simulink model "F_mod_A_mod_gsyn_top_trig_mism_sub_simplified"  (R2022a)
settings: Solver=ode15s  StartTime=0.0  StopTime=10  FixedStep=2.5e-4  MaxStep=5e-2  MinStep=1e-5  RelTol=1e-2  AbsTol=1e-2
model workspace (MAT data in the model file):
  base_gsm = 2.3
  base_gsyn = -2
  cos_amp = 2.5
  cos_center = 0
  friction_factor = 1
  mass_density = 951
  mass_radius = 0.05
  mod_strength_gsm = 1.8
  mod_strength_gsyn = 1.8
  noisePwr = 3e-06
  pendulum_length = 0.4267
  prob_event_loss = 0
  ref_angle = 2
  rel_diff = 0.1
  rel_mod = 100000
  rel_noise = 4
  sampleTime = 0.001
  sin_amp = 2.5
  sin_center = 0
  start_angle = 0
  timescale = 0.004
  torque_max = 0.6
settings Model: SimulationMode=accelerator  Creator=chris  LastModifiedBy=chris
settings SolverCC: MaxConsecutiveZCs=10  MaxConsecutiveMinStep=20  ShapePreserveControl=EnableAll  DecoupledContinuousIntegration=on  MinimalZcImpactIntegration=on
settings DataIOCC: SaveFormat=StructureWithTime
settings OptimizationCC: SimCompilerOptimization=on
settings DebuggingCC: MaxConsecutiveZCsMsg=warning  SolverPrmCheckMsg=warning  ModelReferenceExtraNoncontSigs=warning
settings ModelReferenceCC: ModelReferenceMinAlgLoopOccurrences=on
settings SFSimCC: SimHardwareAcceleration=native
settings ExplorerConfigSet: SimMechanicsOpenEditorOnUpdate=off

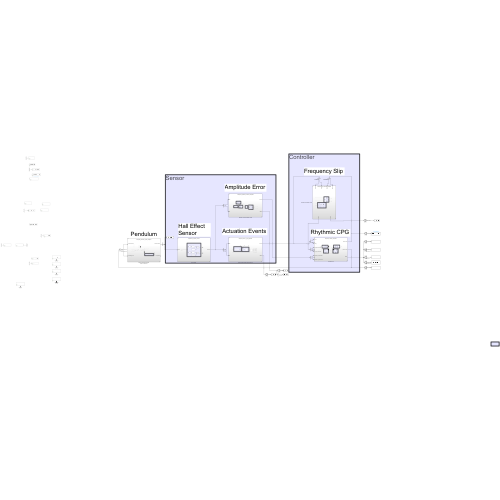
[thumbnail: Simulink's stored preview of the top-level diagram]
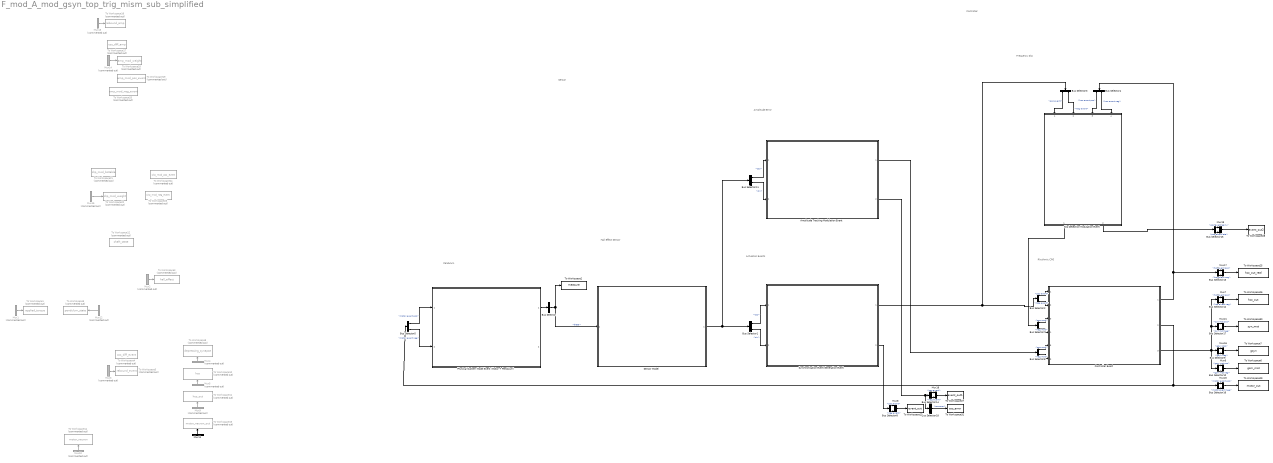
== system F_mod_A_mod_gsyn_top_trig_mism_sub_simplified ==
  note: Controller
  note: Sensor
  note: Pendulum
  note: Hall Effect Sensor
  note: Actuation Events
  note: Amplitude Error
  note: Frequency Slip
  note: Rhythmic CPG
  Amplitude Tracking Modulation Event : Subsystem  VariantControl=Event  ReferencedSubsystem=subsystem_amplitude_modulation_simplified
  Bus Selector : BusSelector  OutputSignals=theta
  Bus Selector1 : BusSelector  OutputSignals=cos,sin
  Bus Selector10 : BusSelector  OutputSignals=gsm mot pos,gsm mot neg
  Bus Selector11 : BusSelector  OutputSignals=cos,sin
  Bus Selector12 : BusSelector  OutputSignals=hco event pos,hco event neg
  Bus Selector13 : BusSelector  OutputSignals=hco event pos,hco event neg
  Bus Selector{2..3,8,14} (4 alike) : BusSelector  OutputSignals=pos event,neg event
  Bus Selector15 : BusSelector  OutputSignals=pos event early,pos event late
  Bus Selector16 : BusSelector  OutputSignals=motor event pos,motor event neg
  Bus Selector17 : BusSelector  OutputSignals=syn mot pos,syn mot neg
  Bus Selector18 : BusSelector  OutputSignals=cos error
  Bus Selector4 : BusSelector  OutputSignals=hco event pos,hco event neg
  Bus Selector5 : BusSelector  OutputSignals=motor event pos,motor event neg
  Bus Selector6 : BusSelector  OutputSignals=pos mod,neg mod
  Bus Selector7 : BusSelector  OutputSignals=pos mod,neg mod
  Bus Selector9 : BusSelector  OutputSignals=gsyn pos,gsyn neg
  Controller Event : Subsystem  VariantControl=Event  ReferencedSubsystem=subsystem_controller_simplified
  Mux{1..5,9..10,13,15} (9 alike) : Mux  Commented=on  Inputs=2
  Mux{6..8,11,16..21} (10 alike) : Mux  Inputs=2
  Mux12 : Mux  Commented=on  Inputs=3
  Mux14 : Mux  Commented=on
  Physical System Model Event (Motor + Pendulum) : Subsystem  VariantControl=Event  ReferencedSubsystem=subsystem_pendulum_system_simplified
  Sensor Model : Subsystem  ReferencedSubsystem=subsystem_hall_effect_encoder
  Slip Detection Modulation Event : Subsystem  VariantControl=Event  ReferencedSubsystem=subsystem_slip_modulation_simplified
  Synchronization Event Generation Event : Subsystem  VariantControl=Event  ReferencedSubsystem=subsystem_event_top_trig_simplified
  To Workspace1 : ToWorkspace  Commented=on  VariableName=applied_torque  SaveFormat=Structure With Time  SampleTime=sampleTime
  To Workspace10 : ToWorkspace  Commented=on  VariableName=hco  SaveFormat=Structure With Time  SampleTime=sampleTime
  To Workspace11 : ToWorkspace  Commented=on  VariableName=hco_out  SaveFormat=Structure With Time  SampleTime=sampleTime
  To Workspace12 : ToWorkspace  Commented=on  VariableName=shaft_state  SaveFormat=Structure With Time  SampleTime=sampleTime
  To Workspace13 : ToWorkspace  VariableName=event_out  SaveFormat=Structure With Time  SampleTime=sampleTime
  To Workspace14 : ToWorkspace  Commented=on  VariableName=motor_neuron  SaveFormat=Structure With Time  SampleTime=sampleTime
  To Workspace15 : ToWorkspace  Commented=on  VariableName=motor_neuron_out  SaveFormat=Structure With Time  SampleTime=sampleTime
  To Workspace16 : ToWorkspace  Commented=on  VariableName=rebound_amp  SaveFormat=Structure With Time  SampleTime=sampleTime
  To Workspace17 : ToWorkspace  Commented=on  VariableName=cos_diff_amp  SaveFormat=Structure With Time  SampleTime=sampleTime
  To Workspace18 : ToWorkspace  Commented=on  VariableName=amp_mod_weight  SaveFormat=Structure With Time  SampleTime=sampleTime
  To Workspace19 : ToWorkspace  Commented=on  VariableName=amp_mod_pos_event  SaveFormat=Structure With Time  SampleTime=sampleTime
  To Workspace2 : ToWorkspace  VariableName=measure  SaveFormat=Structure With Time  SampleTime=sampleTime
  To Workspace20 : ToWorkspace  Commented=on  VariableName=amp_mod_neg_event  SaveFormat=Structure With Time  SampleTime=sampleTime
  To Workspace21 : ToWorkspace  Commented=on  VariableName=slip_mod_bistable  SaveFormat=Structure With Time  SampleTime=sampleTime
  To Workspace22 : ToWorkspace  Commented=on  VariableName=slip_mod_weight  SaveFormat=Structure With Time  SampleTime=sampleTime
  To Workspace23 : ToWorkspace  Commented=on  VariableName=slip_mod_neg_event  SaveFormat=Structure With Time  SampleTime=sampleTime
  To Workspace24 : ToWorkspace  Commented=on  VariableName=slip_mod_pos_event  SaveFormat=Structure With Time  SampleTime=sampleTime
  To Workspace25 : ToWorkspace  VariableName=hco_out_real  SaveFormat=Structure With Time  SampleTime=sampleTime
  To Workspace26 : ToWorkspace  VariableName=hco_out  SaveFormat=Structure With Time  SampleTime=sampleTime
  To Workspace27 : ToWorkspace  VariableName=event_out1  SaveFormat=Structure With Time  SampleTime=sampleTime
  To Workspace28 : ToWorkspace  VariableName=event_out2  SaveFormat=Structure With Time  SampleTime=sampleTime
  To Workspace29 : ToWorkspace  VariableName=motor_out  SaveFormat=Structure With Time  SampleTime=sampleTime
  To Workspace3 : ToWorkspace  Commented=on  VariableName=hall_effect  SaveFormat=Structure With Time  SampleTime=sampleTime
  To Workspace30 : ToWorkspace  VariableName=syn_mot  SaveFormat=Structure With Time  SampleTime=sampleTime
  To Workspace31 : ToWorkspace  VariableName=cos_error  SaveFormat=Structure With Time  SampleTime=sampleTime
  To Workspace4 : ToWorkspace  Commented=on  VariableName=cos_diff_event  SaveFormat=Structure With Time  SampleTime=sampleTime
  To Workspace5 : ToWorkspace  Commented=on  VariableName=rebound_event  SaveFormat=Structure With Time  SampleTime=sampleTime
  To Workspace6 : ToWorkspace  VariableName=gsm_mot  SaveFormat=Structure With Time  SampleTime=sampleTime
  To Workspace7 : ToWorkspace  VariableName=gsyn  SaveFormat=Structure With Time  SampleTime=sampleTime
  To Workspace8 : ToWorkspace  Commented=on  VariableName=depressing_synapse  SaveFormat=Structure With Time  SampleTime=sampleTime
  To Workspace9 : ToWorkspace  Commented=on  VariableName=pendulum_state  SaveFormat=Structure With Time  SampleTime=sampleTime
  wires:
  Mux12/1 -> To Workspace9/1
  Mux1/1 -> To Workspace1/1
  Mux2/1 -> To Workspace3/1
  Sensor Model/1 -> Bus Selector11/1, Bus Selector1/1
  Mux3/1 -> To Workspace5/1
  Mux8/1 -> To Workspace13/1
  Mux4/1 -> To Workspace8/1
  Mux5/1 -> To Workspace10/1
  Mux9/1 -> To Workspace11/1
  Mux10/1 -> To Workspace14/1
  Mux11/1 -> To Workspace15/1
  Mux13/1 -> To Workspace16/1
  Mux14/1 -> To Workspace18/1
  Mux15/1 -> To Workspace22/1
  Bus Selector8/1 -> Mux8/1  "<pos event>"
  Bus Selector8/2 -> Mux8/2  "<neg event>"
  Bus Selector9/2 -> Mux16/2  "<gsyn neg>"
  Bus Selector9/1 -> Mux16/1  "<gsyn pos>"
  Mux16/1 -> To Workspace7/1
  Bus Selector10/2 -> Mux6/2  "<gsm mot neg>"
  Bus Selector10/1 -> Mux6/1  "<gsm mot pos>"
  Mux6/1 -> To Workspace6/1
  Bus Selector/1 -> Sensor Model/1, To Workspace2/1  "<theta>"
  Mux7/1 -> To Workspace26/1
  Bus Selector12/1 -> Mux7/1  "<hco event pos>"
  Bus Selector12/2 -> Mux7/2  "<hco event neg>"
  Bus Selector11/1 -> Amplitude Tracking Modulation Event/1  "<cos>"
  Bus Selector11/2 -> Amplitude Tracking Modulation Event/2  "<sin>"
  Amplitude Tracking Modulation Event/1 -> Bus Selector6/1
  Bus Selector3/1 -> Slip Detection Modulation Event/1  "<pos event>"
  Bus Selector3/2 -> Slip Detection Modulation Event/2  "<neg event>"
  Bus Selector4/1 -> Slip Detection Modulation Event/3  "<hco event pos>"
  Bus Selector4/2 -> Slip Detection Modulation Event/4  "<hco event neg>"
  Slip Detection Modulation Event/1 -> Bus Selector7/1
  Bus Selector1/1 -> Synchronization Event Generation Event/1  "<cos>"
  Bus Selector1/2 -> Synchronization Event Generation Event/2  "<sin>"
  Synchronization Event Generation Event/1 -> Bus Selector3/1, Bus Selector2/1
  Bus Selector2/1 -> Controller Event/1  "<pos event>"
  Bus Selector2/2 -> Controller Event/2  "<neg event>"
  Bus Selector7/1 -> Controller Event/3  "<pos mod>"
  Bus Selector7/2 -> Controller Event/4  "<neg mod>"
  Bus Selector6/1 -> Controller Event/5  "<pos mod>"
  Bus Selector6/2 -> Controller Event/6  "<neg mod>"
  Controller Event/1 -> Bus Selector13/1, Bus Selector4/1
  Controller Event/2 -> Bus Selector16/1, Bus Selector5/1
  Synchronization Event Generation Event/2 -> Bus Selector8/1
  Bus Selector13/2 -> Mux17/2  "<hco event neg>"
  Bus Selector13/1 -> Mux17/1  "<hco event pos>"
  Mux17/1 -> To Workspace25/1
  Bus Selector5/1 -> Physical System Model Event (Motor + Pendulum)/1  "<motor event pos>"
  Bus Selector5/2 -> Physical System Model Event (Motor + Pendulum)/2  "<motor event neg>"
  Physical System Model Event (Motor + Pendulum)/1 -> Bus Selector/1
  Bus Selector14/1 -> Mux18/1  "<pos event>"
  Bus Selector14/2 -> Mux18/2  "<neg event>"
  Mux18/1 -> To Workspace27/1
  Amplitude Tracking Modulation Event/2 -> Bus Selector18/1, Bus Selector14/1
  Bus Selector15/2 -> Mux19/2  "<pos event late>"
  Mux19/1 -> To Workspace28/1
  Slip Detection Modulation Event/2 -> Bus Selector15/1
  Bus Selector15/1 -> Mux19/1  "<pos event early>"
  Mux20/1 -> To Workspace29/1
  Bus Selector16/2 -> Mux20/2  "<motor event neg>"
  Bus Selector16/1 -> Mux20/1  "<motor event pos>"
  Bus Selector17/2 -> Mux21/2  "<syn mot neg>"
  Controller Event/3 -> Bus Selector17/1, Bus Selector12/1, Bus Selector9/1, Bus Selector10/1
  Bus Selector17/1 -> Mux21/1  "<syn mot pos>"
  Mux21/1 -> To Workspace30/1
  Bus Selector18/1 -> To Workspace31/1  "<cos error>"
